simulink model "test_MotionController_v1"  (Simulink 7.6)
settings: Solver=FixedStepDiscrete  StartTime=0.0  StopTime=0  RelTol=1e-3
settings Model: Creator=Administrator  LastModifiedBy=auvt
settings OptimizationCC: InlineParams=on  OptimizeModelRefInitCode=on  LifeSpan=1
settings RTWCC: SystemTargetFile=ert.tlc  GenCodeOnly=on  TemplateMakefile=ert_default_tmf  Description=Real-Time Workshop Embedded Coder  GenerateReport=on  ProcessScript=ert_make_rtw_hook  IncludeHyperlinkInReport=on  LaunchReport=on
settings CodeAppCC: IgnoreCustomStorageClasses=off
settings ERTTargetCC: MultiwordLength=2048  GenerateSampleERTMain=on  IncludeMdlTerminateFcn=off  ERTCustomFileTemplate=example_file_process.tlc  ConvertIfToSwitch=off

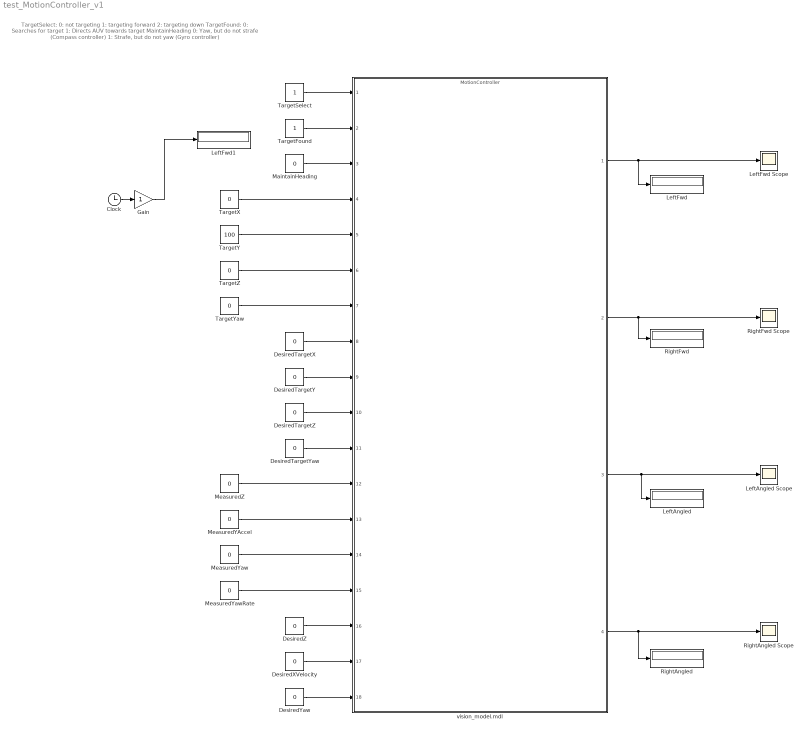
== system test_MotionController_v1 ==
  note: TargetSelect:
      |  0: not targeting
      | 1: targeting forward
      | 2: targeting down
      |
      | TargetFound:
      | 0: Searches for target
      | 1: Directs AUV towards target
      |
      | MaintainHeading
      | 0: Yaw, but do not strafe (Compass controller)
      | 1: Strafe, but do not yaw (Gyro controller)
  Clock : Clock
      settings: Decimation=10
  DesiredTargetX : Constant  Value=0  SampleTime=-1
  DesiredTargetY : Constant  Value=0  SampleTime=-1
  DesiredTargetYaw : Constant  Value=0  SampleTime=-1
  DesiredTargetZ : Constant  Value=0  SampleTime=-1
  DesiredXVelocity : Constant  Value=0  SampleTime=-1
  DesiredYaw : Constant  Value=0  SampleTime=-1
  DesiredZ : Constant  Value=0  SampleTime=-1
  Gain : Gain
  LeftAngled : Display
      settings: Decimation=5
  LeftAngled Scope : Scope
      settings: SaveName=ScopeData2
  LeftFwd : Display
      settings: Decimation=5
  LeftFwd Scope : Scope
      settings: TimeRange=20
  LeftFwd1 : Display
  MaintainHeading : Constant  Value=0  OutDataTypeStr=uint8  SampleTime=-1
  MeasuredYAccel : Constant  Value=0  SampleTime=-1
  MeasuredYaw : Constant  Value=0  SampleTime=-1
  MeasuredYawRate : Constant  Value=0  SampleTime=-1
  MeasuredZ : Constant  Value=0  SampleTime=-1
  RightAngled : Display
      settings: Decimation=5
  RightAngled Scope : Scope
      settings: SaveName=ScopeData3
  RightFwd : Display
      settings: Decimation=5
  RightFwd Scope : Scope
  TargetFound : Constant  SampleTime=-1
  TargetSelect : Constant  SampleTime=-1
  TargetX : Constant  Value=0  SampleTime=-1
  TargetY : Constant  Value=100  SampleTime=-1
  TargetYaw : Constant  Value=0  SampleTime=-1
  TargetZ : Constant  Value=0  SampleTime=-1
  vision_model.mdl : ModelReference  ModelNameDialog=MotionController  SimulationMode=Accelerator  ModelReferenceVersion=1.129  CopyOfModelName=MotionController
  wires:
  TargetSelect/1 -> vision_model.mdl/1
  TargetFound/1 -> vision_model.mdl/2
  MaintainHeading/1 -> vision_model.mdl/3
  TargetX/1 -> vision_model.mdl/4
  TargetY/1 -> vision_model.mdl/5
  TargetZ/1 -> vision_model.mdl/6
  TargetYaw/1 -> vision_model.mdl/7
  DesiredTargetX/1 -> vision_model.mdl/8
  DesiredTargetY/1 -> vision_model.mdl/9
  DesiredTargetZ/1 -> vision_model.mdl/10
  DesiredTargetYaw/1 -> vision_model.mdl/11
  MeasuredZ/1 -> vision_model.mdl/12
  MeasuredYAccel/1 -> vision_model.mdl/13
  MeasuredYawRate/1 -> vision_model.mdl/15
  DesiredZ/1 -> vision_model.mdl/16
  DesiredXVelocity/1 -> vision_model.mdl/17
  DesiredYaw/1 -> vision_model.mdl/18
  vision_model.mdl/1 -> LeftFwd Scope/1, LeftFwd/1
  vision_model.mdl/2 -> RightFwd Scope/1, RightFwd/1
  vision_model.mdl/3 -> LeftAngled Scope/1, LeftAngled/1
  vision_model.mdl/4 -> RightAngled Scope/1, RightAngled/1
  Gain/1 -> LeftFwd1/1
  Clock/1 -> Gain/1
  MeasuredYaw/1 -> vision_model.mdl/14
